simulink model "fsc_model"  (R2015a)
settings: configuration reference "config_cosim" (kept outside this file)
libraries: Sys_CMD x2
settings Model: Creator=ericli  LastModifiedBy=ericli
settings ConfigSetRef: SourceLocation=Base Workspace

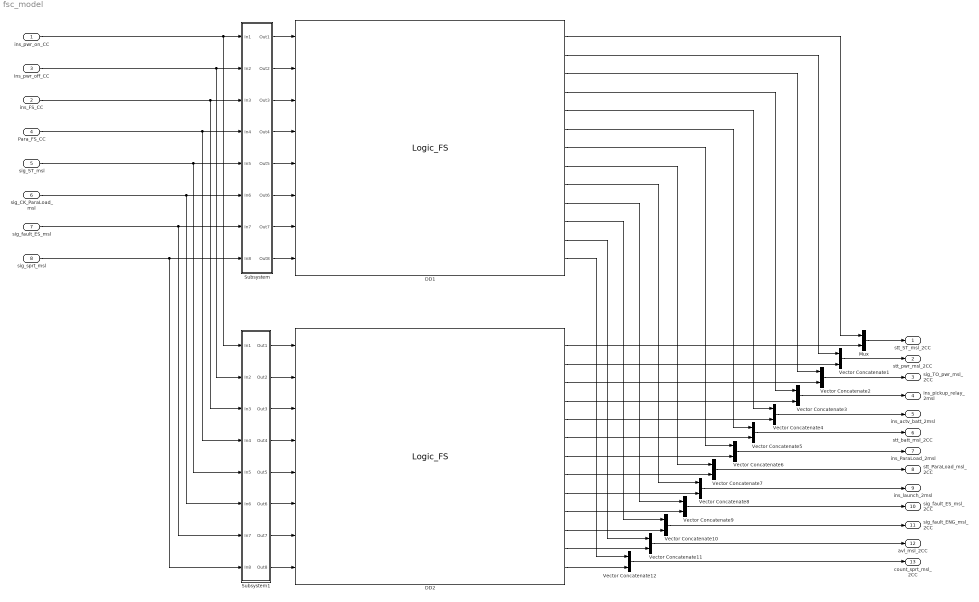
== system fsc_model ==
  ins_pwr_on_CC : Inport  OutDataTypeStr=boolean  PortDimensions=2  SampleTime=[0,1]
  ins_FS_CC : Inport  Port=2  OutDataTypeStr=boolean  PortDimensions=2  SampleTime=[0,1]
  ins_pwr_off_CC : Inport  Port=3  OutDataTypeStr=boolean  PortDimensions=2  SampleTime=[0,1]
  Para_FS_CC : Inport  Port=4  OutDataTypeStr=Bus: BusObject_msg_FSC2msl  PortDimensions=2  SampleTime=[0,1]  BusOutputAsStruct=on
  sig_ST_msl : Inport  Port=5  OutDataTypeStr=boolean  PortDimensions=2  SampleTime=[0,1]
  sig_CK_ParaLoad_msl : Inport  Port=6  OutDataTypeStr=boolean  PortDimensions=2  SampleTime=[0,1]
  sig_fault_ES_msl : Inport  Port=7  OutDataTypeStr=boolean  PortDimensions=2  SampleTime=[0,1]
  sig_sprt_msl : Inport  Port=8  OutDataTypeStr=boolean  PortDimensions=2  SampleTime=[0,1]
  DD1 : Sys_CMD/Logic_FS
  DD2 : Sys_CMD/Logic_FS
  Mux : Mux  Inputs=2
  Subsystem : Subsystem
  Subsystem1 : Subsystem
  Vector Concatenate{1..12} (12 alike) : Concatenate
  stt_ST_msl_2CC : Outport  OutDataTypeStr=boolean  PortDimensions=2  SampleTime=[0,1]
  stt_pwr_msl_2CC : Outport  Port=2  OutDataTypeStr=boolean  PortDimensions=2  SampleTime=[0,1]
  sig_TO_pwr_msl_2CC : Outport  Port=3  OutDataTypeStr=boolean  PortDimensions=2  SampleTime=[0,1]
  ins_pickup_relay_2msl : Outport  Port=4  OutDataTypeStr=boolean  PortDimensions=2  SampleTime=[0,1]
  ins_actv_batt_2msl : Outport  Port=5  OutDataTypeStr=boolean  PortDimensions=2  SampleTime=[0,1]
  stt_batt_msl_2CC : Outport  Port=6  OutDataTypeStr=boolean  PortDimensions=2  SampleTime=[0,1]
  ins_ParaLoad_2msl : Outport  Port=7  OutDataTypeStr=boolean  PortDimensions=2  SampleTime=[0,1]
  stt_ParaLoad_msl_2CC : Outport  Port=8  OutDataTypeStr=boolean  PortDimensions=2  SampleTime=[0,1]
  ins_launch_2msl : Outport  Port=9  OutDataTypeStr=boolean  PortDimensions=2  SampleTime=[0,1]
  sig_fault_ES_msl_2CC : Outport  Port=10  OutDataTypeStr=boolean  PortDimensions=2  SampleTime=[0,1]
  sig_fault_ENG_msl_2CC : Outport  Port=11  OutDataTypeStr=boolean  PortDimensions=2  SampleTime=[0,1]
  avl_msl_2CC : Outport  Port=12  OutDataTypeStr=boolean  PortDimensions=2  SampleTime=[0,1]
  count_sprt_msl_2CC : Outport  Port=13  OutDataTypeStr=double  PortDimensions=2  SampleTime=[0,1]
  wires:
  DD1/4 -> Vector Concatenate3/1
  Subsystem1/8(Out8) -> DD2/8
  DD2/10 -> Vector Concatenate9/2
  Subsystem1/5(Out5) -> DD2/5
  DD1/13 -> Vector Concatenate12/1
  DD2/11 -> Vector Concatenate10/2
  Subsystem/8(Out8) -> DD1/8
  Subsystem/4(Out4) -> DD1/4
  DD2/3 -> Vector Concatenate2/2
  sig_sprt_msl/1 -> Subsystem1/8(In8), Subsystem/8(In8)
  Vector Concatenate2/1 -> sig_TO_pwr_msl_2CC/1
  DD1/2 -> Vector Concatenate1/1
  Subsystem/5(Out5) -> DD1/5
  Vector Concatenate5/1 -> stt_batt_msl_2CC/1
  DD2/2 -> Vector Concatenate1/2
  Vector Concatenate3/1 -> ins_pickup_relay_2msl/1
  Subsystem1/4(Out4) -> DD2/4
  sig_ST_msl/1 -> Subsystem1/5(In5), Subsystem/5(In5)
  DD1/10 -> Vector Concatenate9/1
  DD1/8 -> Vector Concatenate7/1
  Vector Concatenate10/1 -> sig_fault_ENG_msl_2CC/1
  Subsystem1/1(Out1) -> DD2/1
  DD2/1 -> Mux/2
  Vector Concatenate8/1 -> ins_launch_2msl/1
  DD1/3 -> Vector Concatenate2/1
  Vector Concatenate6/1 -> ins_ParaLoad_2msl/1
  Vector Concatenate11/1 -> avl_msl_2CC/1
  Subsystem/7(Out7) -> DD1/7
  Subsystem1/2(Out2) -> DD2/2
  sig_CK_ParaLoad_msl/1 -> Subsystem1/6(In6), Subsystem/6(In6)
  Subsystem/3(Out3) -> DD1/3
  DD1/5 -> Vector Concatenate4/1
  Subsystem1/7(Out7) -> DD2/7
  DD2/7 -> Vector Concatenate6/2
  Vector Concatenate1/1 -> stt_pwr_msl_2CC/1
  Vector Concatenate12/1 -> count_sprt_msl_2CC/1
  ins_pwr_on_CC/1 -> Subsystem1/1(In1), Subsystem/1(In1)
  DD1/11 -> Vector Concatenate10/1
  DD2/12 -> Vector Concatenate11/2
  Vector Concatenate4/1 -> ins_actv_batt_2msl/1
  Subsystem1/3(Out3) -> DD2/3
  DD1/6 -> Vector Concatenate5/1
  DD1/7 -> Vector Concatenate6/1
  DD1/12 -> Vector Concatenate11/1
  Subsystem1/6(Out6) -> DD2/6
  Para_FS_CC/1 -> Subsystem1/4(In4), Subsystem/4(In4)
  ins_FS_CC/1 -> Subsystem1/3(In3), Subsystem/3(In3)
  Mux/1 -> stt_ST_msl_2CC/1
  Vector Concatenate9/1 -> sig_fault_ES_msl_2CC/1
  Vector Concatenate7/1 -> stt_ParaLoad_msl_2CC/1
  DD2/4 -> Vector Concatenate3/2
  ins_pwr_off_CC/1 -> Subsystem1/2(In2), Subsystem/2(In2)
  Subsystem/6(Out6) -> DD1/6
  DD2/8 -> Vector Concatenate7/2
  Subsystem/1(Out1) -> DD1/1
  sig_fault_ES_msl/1 -> Subsystem1/7(In7), Subsystem/7(In7)
  DD2/6 -> Vector Concatenate5/2
  DD2/13 -> Vector Concatenate12/2
  DD1/9 -> Vector Concatenate8/1
  DD2/9 -> Vector Concatenate8/2
  Subsystem/2(Out2) -> DD1/2
  DD1/1 -> Mux/1
  DD2/5 -> Vector Concatenate4/2

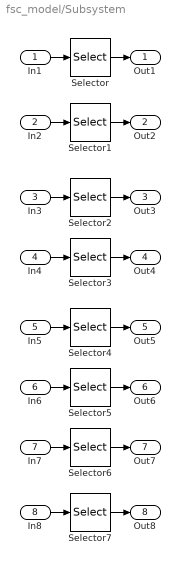
== system fsc_model/Subsystem ==
  In1 : Inport
  In2 : Inport  Port=2
  In3 : Inport  Port=3
  In4 : Inport  Port=4
  In5 : Inport  Port=5
  In6 : Inport  Port=6
  In7 : Inport  Port=7
  In8 : Inport  Port=8
  Selector{,1..7} (8 alike) : Selector  InputPortWidth=2  Indices=[1]
  Out1 : Outport
  Out2 : Outport  Port=2
  Out3 : Outport  Port=3
  Out4 : Outport  Port=4
  Out5 : Outport  Port=5
  Out6 : Outport  Port=6
  Out7 : Outport  Port=7
  Out8 : Outport  Port=8
  wires:
  In1/1 -> Selector/1
  In2/1 -> Selector1/1
  Selector4/1 -> Out5/1
  Selector1/1 -> Out2/1
  Selector6/1 -> Out7/1
  In4/1 -> Selector3/1
  Selector2/1 -> Out3/1
  In8/1 -> Selector7/1
  In5/1 -> Selector4/1
  In3/1 -> Selector2/1
  Selector7/1 -> Out8/1
  In7/1 -> Selector6/1
  Selector/1 -> Out1/1
  Selector5/1 -> Out6/1
  Selector3/1 -> Out4/1
  In6/1 -> Selector5/1

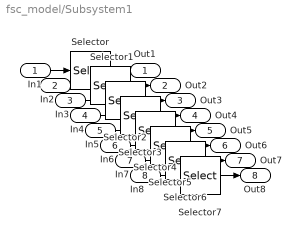
== system fsc_model/Subsystem1 ==
  In1 : Inport
  In2 : Inport  Port=2
  In3 : Inport  Port=3
  In4 : Inport  Port=4
  In5 : Inport  Port=5
  In6 : Inport  Port=6
  In7 : Inport  Port=7
  In8 : Inport  Port=8
  Selector{,1..7} (8 alike) : Selector  InputPortWidth=2  Indices=[2]
  Out1 : Outport
  Out2 : Outport  Port=2
  Out3 : Outport  Port=3
  Out4 : Outport  Port=4
  Out5 : Outport  Port=5
  Out6 : Outport  Port=6
  Out7 : Outport  Port=7
  Out8 : Outport  Port=8
  wires:
  Selector3/1 -> Out4/1
  Selector5/1 -> Out6/1
  Selector2/1 -> Out3/1
  In6/1 -> Selector5/1
  In7/1 -> Selector6/1
  Selector/1 -> Out1/1
  In8/1 -> Selector7/1
  In1/1 -> Selector/1
  Selector6/1 -> Out7/1
  Selector7/1 -> Out8/1
  In4/1 -> Selector3/1
  In5/1 -> Selector4/1
  In2/1 -> Selector1/1
  In3/1 -> Selector2/1
  Selector1/1 -> Out2/1
  Selector4/1 -> Out5/1
